simulink model "environment"  (R2021b)
settings: Solver=VariableStepAuto  StartTime=0.0  StopTime=10.0  RelTol=1e-3
undefined symbols (not defined in the file): Be, Ke, xe
settings Model: Creator=riccardo  LastModifiedBy=riccardo

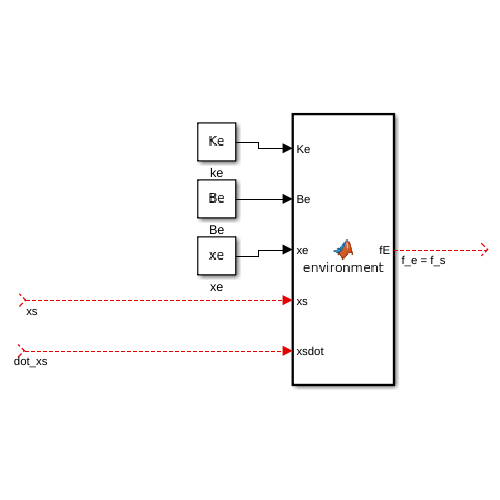
[thumbnail: Simulink's stored preview of the top-level diagram]
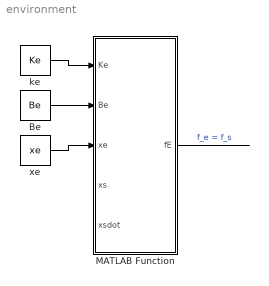
== system environment ==
  Be : Constant  Value=Be
  MATLAB Function : MATLAB Function  TreatAsAtomicUnit=on
  ke : Constant  Value=Ke
  xe : Constant  Value=xe
  wires:
  ke/1 -> MATLAB Function/1(Ke)
  Be/1 -> MATLAB Function/2(Be)
  ? -> MATLAB Function/4(xs)  "xs"
  xe/1 -> MATLAB Function/3(xe)
  ? -> MATLAB Function/5(xsdot)  "dot_xs"
  MATLAB Function/1(fE) -> ?  "f_e = f_s"

== matlab function environment/MATLAB Function ==
  data: Ke input; fE output; Be input; xe input; xs input; xsdot input
function fE = environment(Ke, Be, xe, xs, xsdot)
    if xs > xe
        fE = Ke * (xs - xe) + Be * xsdot; % Plot both contributions Ke and Be
    else
        fE = 0;
    end
end
